simulink model "Linear_Simulation_CTC"  (R2020a)
settings: Solver=ode4  StartTime=0.0  StopTime=25  FixedStep=1e-3  RelTol=1e-3
undefined symbols (not defined in the file): Actc, Bctc, Cctc, K, xs0
settings Model: Creator=Pere Giró  LastModifiedBy=Pere Giró

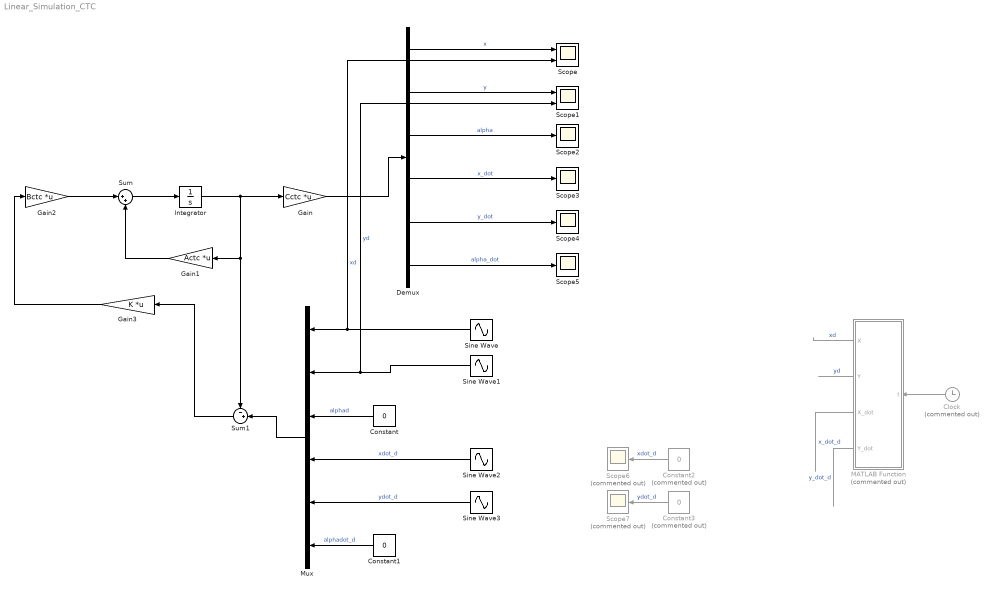
== system Linear_Simulation_CTC ==
  Clock : Clock  Commented=on
  Constant : Constant  Value=0
  Constant1 : Constant  Value=0
  Constant2 : Constant  Commented=on  Value=0
  Constant3 : Constant  Commented=on  Value=0
  Demux : Demux  Outputs=6
  Gain : Gain  Gain=Cctc  Multiplication=Matrix(K*u)
  Gain1 : Gain  Gain=Actc  Multiplication=Matrix(K*u)
  Gain2 : Gain  Gain=Bctc  Multiplication=Matrix(K*u)
  Gain3 : Gain  Gain=K  Multiplication=Matrix(K*u)
  Integrator : Integrator  InitialCondition=xs0
  MATLAB Function : MATLAB Function  Commented=on  TreatAsAtomicUnit=on
  Mux : Mux  Inputs=6
  Scope : Scope  NumInputPorts=2
  Scope1 : Scope  NumInputPorts=2
  Scope{2..5} (4 alike) : Scope
  Scope6 : Scope  Commented=on
  Scope7 : Scope  Commented=on
  Sine Wave : Sin  Frequency=0.3  SampleTime=0
  Sine Wave1 : Sin  Bias=-1  Frequency=0.3  Phase=pi/2  SampleTime=0
  Sine Wave2 : Sin  Amplitude=0.3  Frequency=0.3  Phase=pi/2  SampleTime=0
  Sine Wave3 : Sin  Amplitude=-0.3  Frequency=0.3  SampleTime=0
  Sum : Sum  Inputs=|++
  Sum1 : Sum  Inputs=-+|
  wires:
  Gain2/1 -> Sum/1
  Gain1/1 -> Sum/2
  Sum/1 -> Integrator/1
  Integrator/1 -> Gain1/1, Sum1/1, Gain/1
  Gain/1 -> Demux/1
  Demux/1 -> Scope/1  "x"
  Demux/2 -> Scope1/1  "y"
  Demux/3 -> Scope2/1  "alpha"
  Demux/4 -> Scope3/1  "x_dot"
  Demux/5 -> Scope4/1  "y_dot"
  Demux/6 -> Scope5/1  "alpha_dot"
  Gain3/1 -> Gain2/1
  Sum1/1 -> Gain3/1
  Mux/1 -> Sum1/2
  Sine Wave1/1 -> Mux/2, Scope1/2  "yd"
  Sine Wave/1 -> Scope/2, Mux/1  "xd"
  Constant/1 -> Mux/3  "alphad"
  Sine Wave2/1 -> Mux/4  "xdot_d"
  Sine Wave3/1 -> Mux/5  "ydot_d"
  Constant1/1 -> Mux/6  "alphadot_d"
  Constant2/1 -> Scope6/1  "xdot_d"
  Constant3/1 -> Scope7/1  "ydot_d"
  Clock/1 -> MATLAB Function/1(t)
  MATLAB Function/1(X) -> ?  "xd"
  MATLAB Function/2(Y) -> ?  "yd"
  MATLAB Function/3(X_dot) -> ?  "x_dot_d"
  MATLAB Function/4(Y_dot) -> ?  "y_dot_d"

== matlab function Linear_Simulation_CTC/MATLAB Function ==
  data: t input; X output; Y output; X_dot output; Y_dot output
function [X,Y,X_dot,Y_dot] = fcn(t)

% Polyline Type 2 Square signal
if t <= 5
    X = (1/5)*t;
    Y = 0;
    X_dot = 1/5;
    Y_dot = 0;
elseif t>5 && t<=10
    X = 1;
    Y = (1/5)*(t-5);
    X_dot = 0;
    Y_dot = 1/5;
elseif t>10 && t<=15
    X = (1/5)*(t-10)+1;
    Y = 1;
    X_dot = 1/5;
    Y_dot = 0;
elseif t>15 && t<=20
    X = 2;
    Y = -(1/5)*(t-15)+1;
    X_dot = 0;
    Y_dot = -1/5;
elseif t>20 && t<=25
    X = (1/5)*(t-20)+2;
    Y = 0;
    X_dot = 1/5;
    Y_dot = 0;
else
    X = 3;
    Y = 0;
    X_dot = 0;
    Y_dot = 0;
end
end
